simulink library "speedgoatlib_bce"  (R2024b)
settings: Solver=VariableStepAuto  StartTime=0.0  StopTime=10.0  RelTol=1e-3
undefined symbols (not defined in the file): BCE12, BCE_Set_init, Cell_1, Cell_10, Cell_11, Cell_12, Cell_2, Cell_3, Cell_4, Cell_5, Cell_6, Cell_7, Cell_8, Cell_9, Device_01, FIU12, sg_bce, TSE04
libraries: slrealtimeethercatlib x292, simulink x92, slrealtimeutilitieslib x24
(part 4 of 4)

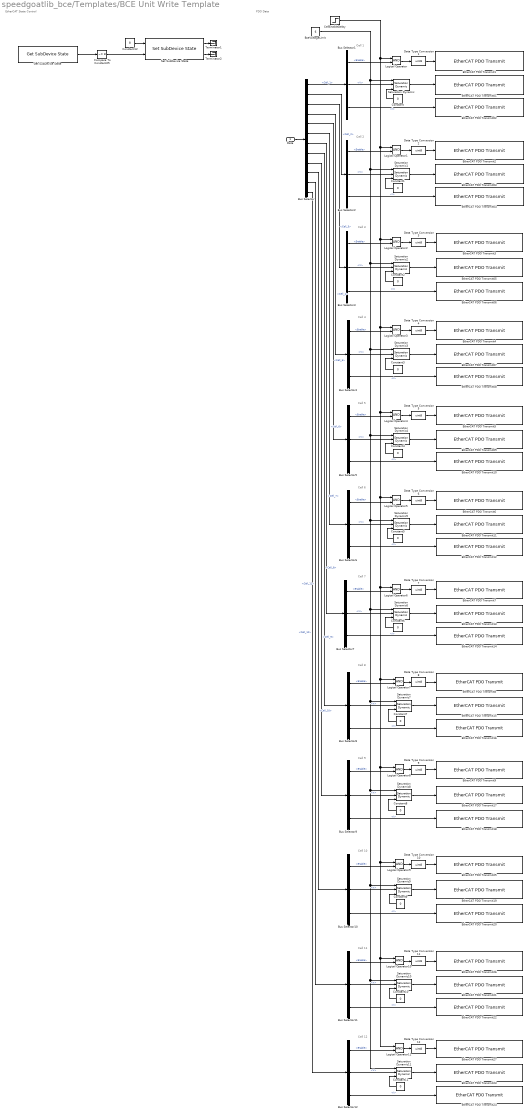
== system speedgoatlib_bce/Templates/BCE Unit Write Template  ==
  note: Cell 2
  note: Cell 12
  note: Cell 11
  note: Cell 6
  note: Cell 10
  note: Cell 3
  note: Cell 5
  note: PDO Data
  note: Cell 7
  note: Cell 1
  note: Cell 9
  note: Cell 8
  note: Cell 4
  note: EtherCAT State Control
  Data : Inport  OutDataTypeStr=Bus: BCE_Set
  BceVoltageLimit : Constant  Value=6
  Bus Selector : BusSelector  OutputSignals=Cell_1,Cell_2,Cell_3,Cell_4,Cell_5,Cell_6,Cell_7,Cell_8,Cell_9,Cell_10,Cell_11,Cell_12
  Bus Selector{1..12} (12 alike) : BusSelector  OutputSignals=Enable,V,I
  CellEnableDelay : Step  Time=2  SampleTime=0
  Compare To Constant25 : simulink/Logic and Bit Operations/Compare To Constant  relop=~=  const=8  OutDataTypeStr=boolean
  Constant{,1..11} (12 alike) : Constant  Value=0
  Constant12 : Constant  Value=8  OutDataTypeStr=int32
  Data Type Conversion{1..12} (12 alike) : DataTypeConversion  OutDataTypeStr=uint8  SaturateOnIntegerOverflow=off  RndMeth=Floor
  EtherCAT PDO Transmit01 : slrealtimeethercatlib/EtherCAT PDO Transmit  Priority=3  sig_name=Device_01 (BCE12-0605).Rx_Cell_01.setVoltage  sig_offset=8  sig_type=single  type_size=32  sig_dim=1  device_id=0  sample_time=0.001000
  EtherCAT PDO Transmit02 : slrealtimeethercatlib/EtherCAT PDO Transmit  Priority=3  sig_name=Device_01 (BCE12-0605).Rx_Cell_01.setCurrent  sig_offset=40  sig_type=single  type_size=32  sig_dim=1  device_id=0  sample_time=0.001000
  EtherCAT PDO Transmit03 : slrealtimeethercatlib/EtherCAT PDO Transmit  Priority=3  sig_name=Device_01 (BCE12-0605).Rx_Cell_02.setVoltage  sig_offset=80  sig_type=single  type_size=32  sig_dim=1  device_id=0  sample_time=0.001000
  EtherCAT PDO Transmit04 : slrealtimeethercatlib/EtherCAT PDO Transmit  Priority=3  sig_name=Device_01 (BCE12-0605).Rx_Cell_02.setCurrent  sig_offset=112  sig_type=single  type_size=32  sig_dim=1  device_id=0  sample_time=0.001000
  EtherCAT PDO Transmit05 : slrealtimeethercatlib/EtherCAT PDO Transmit  Priority=3  sig_name=Device_01 (BCE12-0605).Rx_Cell_03.setVoltage  sig_offset=152  sig_type=single  type_size=32  sig_dim=1  device_id=0  sample_time=0.001000
  EtherCAT PDO Transmit06 : slrealtimeethercatlib/EtherCAT PDO Transmit  Priority=3  sig_name=Device_01 (BCE12-0605).Rx_Cell_03.setCurrent  sig_offset=184  sig_type=single  type_size=32  sig_dim=1  device_id=0  sample_time=0.001000
  EtherCAT PDO Transmit07 : slrealtimeethercatlib/EtherCAT PDO Transmit  Priority=3  sig_name=Device_01 (BCE12-0605).Rx_Cell_04.setVoltage  sig_offset=224  sig_type=single  type_size=32  sig_dim=1  device_id=0  sample_time=0.001000
  EtherCAT PDO Transmit08 : slrealtimeethercatlib/EtherCAT PDO Transmit  Priority=3  sig_name=Device_01 (BCE12-0605).Rx_Cell_04.setCurrent  sig_offset=256  sig_type=single  type_size=32  sig_dim=1  device_id=0  sample_time=0.001000
  EtherCAT PDO Transmit09 : slrealtimeethercatlib/EtherCAT PDO Transmit  Priority=3  sig_name=Device_01 (BCE12-0605).Rx_Cell_05.setVoltage  sig_offset=296  sig_type=single  type_size=32  sig_dim=1  device_id=0  sample_time=0.001000
  EtherCAT PDO Transmit1 : slrealtimeethercatlib/EtherCAT PDO Transmit  Priority=3  sig_name=Device_01 (BCE12-0605).Rx_Cell_01.enableCell  sig_offset=0  sig_type=uint8  type_size=8  sig_dim=1  device_id=0  sample_time=0.001000
  EtherCAT PDO Transmit10 : slrealtimeethercatlib/EtherCAT PDO Transmit  Priority=3  sig_name=Device_01 (BCE12-0605).Rx_Cell_05.setCurrent  sig_offset=328  sig_type=single  type_size=32  sig_dim=1  device_id=0  sample_time=0.001000
  EtherCAT PDO Transmit11 : slrealtimeethercatlib/EtherCAT PDO Transmit  Priority=3  sig_name=Device_01 (BCE12-0605).Rx_Cell_06.setVoltage  sig_offset=368  sig_type=single  type_size=32  sig_dim=1  device_id=0  sample_time=0.001000
  EtherCAT PDO Transmit12 : slrealtimeethercatlib/EtherCAT PDO Transmit  Priority=3  sig_name=Device_01 (BCE12-0605).Rx_Cell_06.setCurrent  sig_offset=400  sig_type=single  type_size=32  sig_dim=1  device_id=0  sample_time=0.001000
  EtherCAT PDO Transmit13 : slrealtimeethercatlib/EtherCAT PDO Transmit  Priority=3  sig_name=Device_01 (BCE12-0605).Rx_Cell_07.setVoltage  sig_offset=440  sig_type=single  type_size=32  sig_dim=1  device_id=0  sample_time=0.001000
  EtherCAT PDO Transmit14 : slrealtimeethercatlib/EtherCAT PDO Transmit  Priority=3  sig_name=Device_01 (BCE12-0605).Rx_Cell_07.setCurrent  sig_offset=472  sig_type=single  type_size=32  sig_dim=1  device_id=0  sample_time=0.001000
  EtherCAT PDO Transmit15 : slrealtimeethercatlib/EtherCAT PDO Transmit  Priority=3  sig_name=Device_01 (BCE12-0605).Rx_Cell_08.setVoltage  sig_offset=512  sig_type=single  type_size=32  sig_dim=1  device_id=0  sample_time=0.001000
  EtherCAT PDO Transmit16 : slrealtimeethercatlib/EtherCAT PDO Transmit  Priority=3  sig_name=Device_01 (BCE12-0605).Rx_Cell_08.setCurrent  sig_offset=544  sig_type=single  type_size=32  sig_dim=1  device_id=0  sample_time=0.001000
  EtherCAT PDO Transmit17 : slrealtimeethercatlib/EtherCAT PDO Transmit  Priority=3  sig_name=Device_01 (BCE12-0605).Rx_Cell_09.setVoltage  sig_offset=584  sig_type=single  type_size=32  sig_dim=1  device_id=0  sample_time=0.001000
  EtherCAT PDO Transmit18 : slrealtimeethercatlib/EtherCAT PDO Transmit  Priority=3  sig_name=Device_01 (BCE12-0605).Rx_Cell_09.setCurrent  sig_offset=616  sig_type=single  type_size=32  sig_dim=1  device_id=0  sample_time=0.001000
  EtherCAT PDO Transmit19 : slrealtimeethercatlib/EtherCAT PDO Transmit  Priority=3  sig_name=Device_01 (BCE12-0605).Rx_Cell_10.setVoltage  sig_offset=656  sig_type=single  type_size=32  sig_dim=1  device_id=0  sample_time=0.001000
  EtherCAT PDO Transmit2 : slrealtimeethercatlib/EtherCAT PDO Transmit  Priority=3  sig_name=Device_01 (BCE12-0605).Rx_Cell_02.enableCell  sig_offset=72  sig_type=uint8  type_size=8  sig_dim=1  device_id=0  sample_time=0.001000
  EtherCAT PDO Transmit20 : slrealtimeethercatlib/EtherCAT PDO Transmit  Priority=3  sig_name=Device_01 (BCE12-0605).Rx_Cell_10.setCurrent  sig_offset=688  sig_type=single  type_size=32  sig_dim=1  device_id=0  sample_time=0.001000
  EtherCAT PDO Transmit21 : slrealtimeethercatlib/EtherCAT PDO Transmit  Priority=3  sig_name=Device_01 (BCE12-0605).Rx_Cell_11.setVoltage  sig_offset=728  sig_type=single  type_size=32  sig_dim=1  device_id=0  sample_time=0.001000
  EtherCAT PDO Transmit22 : slrealtimeethercatlib/EtherCAT PDO Transmit  Priority=3  sig_name=Device_01 (BCE12-0605).Rx_Cell_11.setCurrent  sig_offset=760  sig_type=single  type_size=32  sig_dim=1  device_id=0  sample_time=0.001000
  EtherCAT PDO Transmit23 : slrealtimeethercatlib/EtherCAT PDO Transmit  Priority=3  sig_name=Device_01 (BCE12-0605).Rx_Cell_12.setVoltage  sig_offset=800  sig_type=single  type_size=32  sig_dim=1  device_id=0  sample_time=0.001000
  EtherCAT PDO Transmit24 : slrealtimeethercatlib/EtherCAT PDO Transmit  Priority=3  sig_name=Device_01 (BCE12-0605).Rx_Cell_12.setCurrent  sig_offset=832  sig_type=single  type_size=32  sig_dim=1  device_id=0  sample_time=0.001000
  EtherCAT PDO Transmit25 : slrealtimeethercatlib/EtherCAT PDO Transmit  Priority=3  sig_name=Device_01 (BCE12-0605).Rx_Cell_10.enableCell  sig_offset=648  sig_type=uint8  type_size=8  sig_dim=1  device_id=0  sample_time=0.001000
  EtherCAT PDO Transmit26 : slrealtimeethercatlib/EtherCAT PDO Transmit  Priority=3  sig_name=Device_01 (BCE12-0605).Rx_Cell_11.enableCell  sig_offset=720  sig_type=uint8  type_size=8  sig_dim=1  device_id=0  sample_time=0.001000
  EtherCAT PDO Transmit27 : slrealtimeethercatlib/EtherCAT PDO Transmit  Priority=3  sig_name=Device_01 (BCE12-0605).Rx_Cell_12.enableCell  sig_offset=792  sig_type=uint8  type_size=8  sig_dim=1  device_id=0  sample_time=0.001000
  EtherCAT PDO Transmit3 : slrealtimeethercatlib/EtherCAT PDO Transmit  Priority=3  sig_name=Device_01 (BCE12-0605).Rx_Cell_03.enableCell  sig_offset=144  sig_type=uint8  type_size=8  sig_dim=1  device_id=0  sample_time=0.001000
  EtherCAT PDO Transmit4 : slrealtimeethercatlib/EtherCAT PDO Transmit  Priority=3  sig_name=Device_01 (BCE12-0605).Rx_Cell_04.enableCell  sig_offset=216  sig_type=uint8  type_size=8  sig_dim=1  device_id=0  sample_time=0.001000
  EtherCAT PDO Transmit5 : slrealtimeethercatlib/EtherCAT PDO Transmit  Priority=3  sig_name=Device_01 (BCE12-0605).Rx_Cell_05.enableCell  sig_offset=288  sig_type=uint8  type_size=8  sig_dim=1  device_id=0  sample_time=0.001000
  EtherCAT PDO Transmit6 : slrealtimeethercatlib/EtherCAT PDO Transmit  Priority=3  sig_name=Device_01 (BCE12-0605).Rx_Cell_06.enableCell  sig_offset=360  sig_type=uint8  type_size=8  sig_dim=1  device_id=0  sample_time=0.001000
  EtherCAT PDO Transmit7 : slrealtimeethercatlib/EtherCAT PDO Transmit  Priority=3  sig_name=Device_01 (BCE12-0605).Rx_Cell_07.enableCell  sig_offset=432  sig_type=uint8  type_size=8  sig_dim=1  device_id=0  sample_time=0.001000
  EtherCAT PDO Transmit8 : slrealtimeethercatlib/EtherCAT PDO Transmit  Priority=3  sig_name=Device_01 (BCE12-0605).Rx_Cell_08.enableCell  sig_offset=504  sig_type=uint8  type_size=8  sig_dim=1  device_id=0  sample_time=0.001000
  EtherCAT PDO Transmit9 : slrealtimeethercatlib/EtherCAT PDO Transmit  Priority=3  sig_name=Device_01 (BCE12-0605).Rx_Cell_09.enableCell  sig_offset=576  sig_type=uint8  type_size=8  sig_dim=1  device_id=0  sample_time=0.001000
  Get SubDevice State : slrealtimeethercatlib/Get SubDevice State  device_id=0  sample_time=1  subdevice_addr=0  selected_subdevice=Term 1 (EK1100)  timeout=500  subdevice_found=0
  Logical Operator{,1..11} (12 alike) : Logic  AllPortsSameDT=off  OutDataTypeStr=boolean
  Saturation Dynamic{,1..11} (12 alike) : simulink/Discontinuities/Saturation Dynamic  OutMin=[]  OutMax=[]  OutDataTypeStr=Inherit: Same as second input  OutDataType=fixdt(1, 16)  OutScaling=2^-10  DoSatur=off
  Set SubDevice State : slrealtimeethercatlib/Set SubDevice State  device_id=0  sample_time=1  subdevice_addr=0  selected_subdevice=Term 1 (EK1100)  subdevice_found=0
  Terminator1 : Terminator
  Terminator2 : Terminator
  wires:
  Data Type Conversion8/1 -> EtherCAT PDO Transmit8/1
  Bus Selector9/2 -> Saturation Dynamic8/2  "<V>"
  Bus Selector12/2 -> Saturation Dynamic11/2  "<V>"
  Bus Selector2/2 -> Saturation Dynamic1/2  "<V>"
  Bus Selector/7 -> Bus Selector7/1  "<Cell_7>"
  Bus Selector11/2 -> Saturation Dynamic10/2  "<V>"
  Bus Selector/1 -> Bus Selector1/1  "<Cell_1>"
  Bus Selector8/3 -> EtherCAT PDO Transmit16/1  "<I>"
  Bus Selector/3 -> Bus Selector3/1  "<Cell_3>"
  Bus Selector1/2 -> Saturation Dynamic/2  "<V>"
  Bus Selector/2 -> Bus Selector2/1  "<Cell_2>"
  Bus Selector/6 -> Bus Selector6/1  "<Cell_6>"
  Data Type Conversion2/1 -> EtherCAT PDO Transmit2/1
  Bus Selector7/2 -> Saturation Dynamic6/2  "<V>"
  Bus Selector7/3 -> EtherCAT PDO Transmit14/1  "<I>"
  Bus Selector/9 -> Bus Selector9/1  "<Cell_9>"
  Data Type Conversion4/1 -> EtherCAT PDO Transmit4/1
  Data Type Conversion6/1 -> EtherCAT PDO Transmit6/1
  Data Type Conversion9/1 -> EtherCAT PDO Transmit9/1
  Data Type Conversion5/1 -> EtherCAT PDO Transmit5/1
  Data Type Conversion12/1 -> EtherCAT PDO Transmit27/1
  Data Type Conversion10/1 -> EtherCAT PDO Transmit25/1
  Data Type Conversion1/1 -> EtherCAT PDO Transmit1/1
  Bus Selector4/3 -> EtherCAT PDO Transmit08/1  "<I>"
  Bus Selector/12 -> Bus Selector12/1  "<Cell_12>"
  Bus Selector3/3 -> EtherCAT PDO Transmit06/1  "<I>"
  Bus Selector6/2 -> Saturation Dynamic5/2  "<V>"
  Bus Selector4/2 -> Saturation Dynamic3/2  "<V>"
  Data Type Conversion3/1 -> EtherCAT PDO Transmit3/1
  Bus Selector1/3 -> EtherCAT PDO Transmit02/1  "<I>"
  Bus Selector/10 -> Bus Selector10/1  "<Cell_10>"
  Bus Selector/5 -> Bus Selector5/1  "<Cell_5>"
  Bus Selector12/3 -> EtherCAT PDO Transmit24/1  "<I>"
  Bus Selector10/2 -> Saturation Dynamic9/2  "<V>"
  Bus Selector2/3 -> EtherCAT PDO Transmit04/1  "<I>"
  Bus Selector3/2 -> Saturation Dynamic2/2  "<V>"
  Bus Selector/11 -> Bus Selector11/1  "<Cell_11>"
  Bus Selector10/3 -> EtherCAT PDO Transmit20/1  "<I>"
  Data/1 -> Bus Selector/1
  Bus Selector5/3 -> EtherCAT PDO Transmit10/1  "<I>"
  Data Type Conversion11/1 -> EtherCAT PDO Transmit26/1
  Bus Selector5/2 -> Saturation Dynamic4/2  "<V>"
  Bus Selector8/2 -> Saturation Dynamic7/2  "<V>"
  Bus Selector/8 -> Bus Selector8/1  "<Cell_8>"
  Bus Selector9/3 -> EtherCAT PDO Transmit18/1  "<I>"
  Bus Selector11/3 -> EtherCAT PDO Transmit22/1  "<I>"
  Data Type Conversion7/1 -> EtherCAT PDO Transmit7/1
  Bus Selector/4 -> Bus Selector4/1  "<Cell_4>"
  Bus Selector6/3 -> EtherCAT PDO Transmit12/1  "<I>"
  Saturation Dynamic/1 -> EtherCAT PDO Transmit01/1
  Constant/1 -> Saturation Dynamic/3
  BceVoltageLimit/1 -> Saturation Dynamic/1, Saturation Dynamic11/1, Saturation Dynamic10/1, Saturation Dynamic9/1, Saturation Dynamic8/1, Saturation Dynamic7/1, Saturation Dynamic6/1, Saturation Dynamic5/1, Saturation Dynamic4/1, Saturation Dynamic3/1, Saturation Dynamic2/1, Saturation Dynamic1/1
  Constant1/1 -> Saturation Dynamic1/3
  Saturation Dynamic1/1 -> EtherCAT PDO Transmit03/1
  Constant2/1 -> Saturation Dynamic2/3
  Saturation Dynamic2/1 -> EtherCAT PDO Transmit05/1
  Constant3/1 -> Saturation Dynamic3/3
  Saturation Dynamic3/1 -> EtherCAT PDO Transmit07/1
  Constant4/1 -> Saturation Dynamic4/3
  Saturation Dynamic4/1 -> EtherCAT PDO Transmit09/1
  Constant5/1 -> Saturation Dynamic5/3
  Saturation Dynamic5/1 -> EtherCAT PDO Transmit11/1
  Constant6/1 -> Saturation Dynamic6/3
  Saturation Dynamic6/1 -> EtherCAT PDO Transmit13/1
  Constant7/1 -> Saturation Dynamic7/3
  Saturation Dynamic7/1 -> EtherCAT PDO Transmit15/1
  Constant8/1 -> Saturation Dynamic8/3
  Saturation Dynamic8/1 -> EtherCAT PDO Transmit17/1
  Constant9/1 -> Saturation Dynamic9/3
  Saturation Dynamic9/1 -> EtherCAT PDO Transmit19/1
  Constant10/1 -> Saturation Dynamic10/3
  Saturation Dynamic10/1 -> EtherCAT PDO Transmit21/1
  Constant11/1 -> Saturation Dynamic11/3
  Saturation Dynamic11/1 -> EtherCAT PDO Transmit23/1
  Get SubDevice State/1 -> Compare To Constant25/1
  Set SubDevice State/2 -> Terminator2/1
  Set SubDevice State/1 -> Terminator1/1
  Compare To Constant25/1 -> Set SubDevice State/2
  Constant12/1 -> Set SubDevice State/1
  CellEnableDelay/1 -> Logical Operator11/1, Logical Operator10/1, Logical Operator9/1, Logical Operator8/1, Logical Operator7/1, Logical Operator6/1, Logical Operator5/1, Logical Operator4/1, Logical Operator3/1, Logical Operator2/1, Logical Operator1/1, Logical Operator/1
  Bus Selector1/1 -> Logical Operator/2  "<Enable>"
  Logical Operator/1 -> Data Type Conversion1/1
  Bus Selector2/1 -> Logical Operator1/2  "<Enable>"
  Logical Operator1/1 -> Data Type Conversion2/1
  Bus Selector3/1 -> Logical Operator2/2  "<Enable>"
  Logical Operator2/1 -> Data Type Conversion3/1
  Bus Selector4/1 -> Logical Operator3/2  "<Enable>"
  Logical Operator3/1 -> Data Type Conversion4/1
  Bus Selector5/1 -> Logical Operator4/2  "<Enable>"
  Logical Operator4/1 -> Data Type Conversion5/1
  Bus Selector6/1 -> Logical Operator5/2  "<Enable>"
  Logical Operator5/1 -> Data Type Conversion6/1
  Bus Selector7/1 -> Logical Operator6/2  "<Enable>"
  Logical Operator6/1 -> Data Type Conversion7/1
  Bus Selector8/1 -> Logical Operator7/2  "<Enable>"
  Logical Operator7/1 -> Data Type Conversion8/1
  Bus Selector9/1 -> Logical Operator8/2  "<Enable>"
  Logical Operator8/1 -> Data Type Conversion9/1
  Bus Selector10/1 -> Logical Operator9/2  "<Enable>"
  Logical Operator9/1 -> Data Type Conversion10/1
  Bus Selector11/1 -> Logical Operator10/2  "<Enable>"
  Logical Operator10/1 -> Data Type Conversion11/1
  Bus Selector12/1 -> Logical Operator11/2  "<Enable>"
  Logical Operator11/1 -> Data Type Conversion12/1

== system speedgoatlib_bce/Templates/FIU Channel Read Template  ==
  note: Channel X
  Bus Creator : BusCreator  Inputs=1  OutDataTypeStr=Bus: FIU_Get
      settings: InheritFromInputs=off
  EtherCAT PDO Receive01 : slrealtimeethercatlib/EtherCAT PDO Receive  Priority=2  sig_name=Device_01 (FIU12-1).Tx_Channel_01.status  sig_offset=0  sig_type=uint8  type_size=8  sig_dim=1  device_id=0  sample_time=0.001000
  Data : Outport  OutDataTypeStr=Bus: FIU_Get
  wires:
  EtherCAT PDO Receive01/1 -> Bus Creator/1  "ChX_Status"
  Bus Creator/1 -> Data/1

== system speedgoatlib_bce/Templates/FIU Channel Write Template  ==
  note: Update
  Data : Inport  OutDataTypeStr=Bus: FIU_Set
  Add : Sum  Inputs=+++
  Bus Selector : BusSelector  OutputSignals=FaultState,SensePlusBroken,SenseMinusBroken
  Constant3 : Constant  Value=8  OutDataTypeStr=uint8
  Constant4 : Constant  Value=0  OutDataTypeStr=uint8
  Constant6 : Constant  Value=16  OutDataTypeStr=uint8
  Constant7 : Constant  Value=0  OutDataTypeStr=uint8
  EtherCAT PDO Transmit02 : slrealtimeethercatlib/EtherCAT PDO Transmit  Priority=3  sig_name=Device_01 (FIU12-1).Rx_Channel_01.faultState  sig_offset=8  sig_type=uint8  type_size=8  sig_dim=1  device_id=0  sample_time=0.001000
  EtherCAT State Control : Subsystem
  Range Assert : MATLAB Function  TreatAsAtomicUnit=on
  Switch : Switch  Criteria=u2 > Threshold  SaturateOnIntegerOverflow=off  InputSameDT=off
  Switch1 : Switch  Criteria=u2 > Threshold  SaturateOnIntegerOverflow=off  InputSameDT=off
  wires:
  Bus Selector/1 -> Range Assert/1(u)  "<FaultState>"
  Switch1/1 -> Add/3
  Bus Selector/3 -> Switch1/2  "<SenseMinusBroken>"
  Add/1 -> EtherCAT PDO Transmit02/1
  Constant7/1 -> Switch1/3
  Constant4/1 -> Switch/3
  Switch/1 -> Add/2
  Constant3/1 -> Switch/1
  Constant6/1 -> Switch1/1
  Bus Selector/2 -> Switch/2  "<SensePlusBroken>"
  Data/1 -> Bus Selector/1
  Range Assert/1(y) -> Add/1

== system speedgoatlib_bce/Templates/TSE Channel Read Template  ==
  note: Channel X
  Bus Creator : BusCreator  Inputs=1  OutDataTypeStr=Bus: TSE_Get
      settings: InheritFromInputs=off
  EtherCAT PDO Receive01 : slrealtimeethercatlib/EtherCAT PDO Receive  Priority=2  sig_name=Device_01 (TSE04-1000-1).Tx_Channel_01.status  sig_offset=0  sig_type=single  type_size=32  sig_dim=1  device_id=0  sample_time=0.001000
  Data : Outport  OutDataTypeStr=Bus: TSE_Get
  wires:
  EtherCAT PDO Receive01/1 -> Bus Creator/1  "ChX_Status"
  Bus Creator/1 -> Data/1

== system speedgoatlib_bce/Templates/TSE Channel Write Template  ==
  note: Update
  Data : Inport  OutDataTypeStr=Bus: TSE_Set
  Bus Selector : BusSelector  OutputSignals=Resistance
  EtherCAT PDO Transmit02 : slrealtimeethercatlib/EtherCAT PDO Transmit  Priority=3  sig_name=Device_01 (TSE04-1000-1).Rx_Channel_01.resistance  sig_offset=8  sig_type=double  type_size=64  sig_dim=1  device_id=0  sample_time=0.001000
  EtherCAT State Control : Subsystem
  wires:
  Data/1 -> Bus Selector/1
  Bus Selector/1 -> EtherCAT PDO Transmit02/1  "<Resistance>"

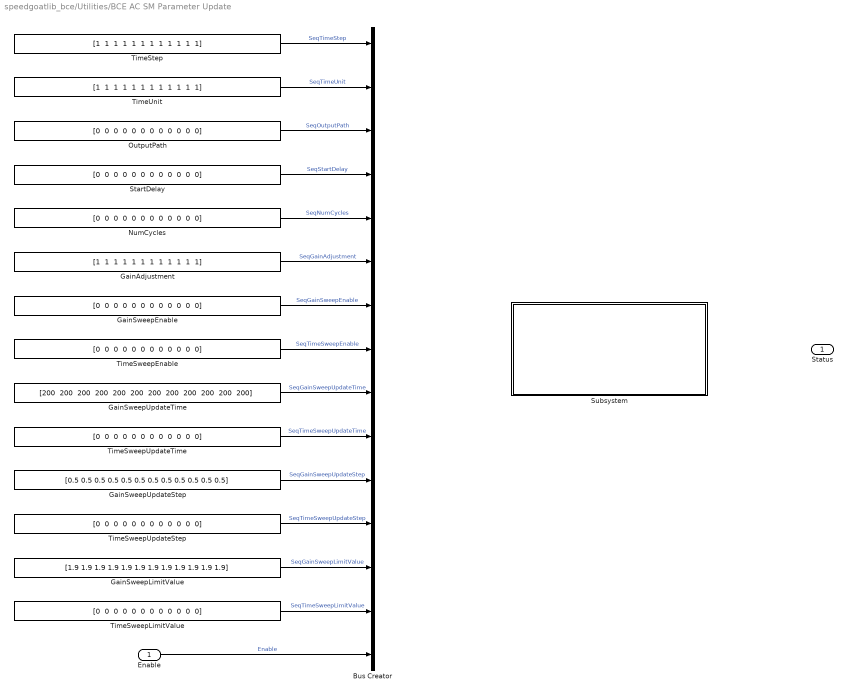
== system speedgoatlib_bce/Utilities/BCE AC SM Parameter Update  ==
  Enable : Inport  OutDataTypeStr=boolean
  Bus Creator : BusCreator  Inputs=15
  GainAdjustment : Constant  Value="[1  1  1  1  1  1  1  1  1  1  1  1]"  OutDataTypeStr=double
  GainSweepEnable : Constant  Value="[0  0  0  0  0  0  0  0  0  0  0  0]"  OutDataTypeStr=boolean
  GainSweepLimitValue : Constant  Value="[1.9         1.9         1.9         1.9         1.9         1.9         1.9         1.9         1.9         1.9         1.9         1.9]"  OutDataTypeStr=double
  GainSweepUpdateStep : Constant  Value="[0.5         0.5         0.5         0.5         0.5         0.5         0.5         0.5         0.5         0.5         0.5         0.5]"  OutDataTypeStr=double
  GainSweepUpdateTime : Constant  Value="[200  200  200  200  200  200  200  200  200  200  200  200]"  OutDataTypeStr=uint16
  NumCycles : Constant  Value="[0  0  0  0  0  0  0  0  0  0  0  0]"  OutDataTypeStr=uint16
  OutputPath : Constant  Value="[0  0  0  0  0  0  0  0  0  0  0  0]"  OutDataTypeStr=boolean
  StartDelay : Constant  Value="[0  0  0  0  0  0  0  0  0  0  0  0]"  OutDataTypeStr=uint16
  Subsystem : Subsystem
  TimeStep : Constant  Value="[1  1  1  1  1  1  1  1  1  1  1  1]"  OutDataTypeStr=uint16
  TimeSweepEnable : Constant  Value="[0  0  0  0  0  0  0  0  0  0  0  0]"  OutDataTypeStr=boolean
  TimeSweepLimitValue : Constant  Value="[0  0  0  0  0  0  0  0  0  0  0  0]"  OutDataTypeStr=uint16
  TimeSweepUpdateStep : Constant  Value="[0  0  0  0  0  0  0  0  0  0  0  0]"  OutDataTypeStr=uint16
  TimeSweepUpdateTime : Constant  Value="[0  0  0  0  0  0  0  0  0  0  0  0]"  OutDataTypeStr=uint16
  TimeUnit : Constant  Value="[1  1  1  1  1  1  1  1  1  1  1  1]"  OutDataTypeStr=boolean
  Status : Outport
  wires:
  GainSweepLimitValue/1 -> Bus Creator/13  "SeqGainSweepLimitValue"
  TimeSweepUpdateStep/1 -> Bus Creator/12  "SeqTimeSweepUpdateStep"
  GainSweepUpdateStep/1 -> Bus Creator/11  "SeqGainSweepUpdateStep"
  TimeSweepLimitValue/1 -> Bus Creator/14  "SeqTimeSweepLimitValue"
  TimeSweepUpdateTime/1 -> Bus Creator/10  "SeqTimeSweepUpdateTime"
  GainSweepUpdateTime/1 -> Bus Creator/9  "SeqGainSweepUpdateTime"
  TimeStep/1 -> Bus Creator/1  "SeqTimeStep"
  OutputPath/1 -> Bus Creator/3  "SeqOutputPath"
  TimeSweepEnable/1 -> Bus Creator/8  "SeqTimeSweepEnable"
  StartDelay/1 -> Bus Creator/4  "SeqStartDelay"
  GainSweepEnable/1 -> Bus Creator/7  "SeqGainSweepEnable"
  TimeUnit/1 -> Bus Creator/2  "SeqTimeUnit"
  NumCycles/1 -> Bus Creator/5  "SeqNumCycles"
  GainAdjustment/1 -> Bus Creator/6  "SeqGainAdjustment"
  Enable/1 -> Bus Creator/15  "Enable"

== system speedgoatlib_bce/Utilities/BMTS Bus Pack  ==
  Cell_1.Enable : Inport
  Cell_2.Enable : Inport  Port=2
  Cell_1.V : Inport  Port=3
  Cell_2.V : Inport  Port=4
  Cell_1.I : Inport  Port=5
  Cell_2.I : Inport  Port=6
  Bus Assignment : BusAssignment  AssignedSignals=Cell_1.Enable,Cell_2.Enable,Cell_1.V,Cell_2.V,Cell_1.I,Cell_2.I
  Bus Structure : Constant  Value=BCE_Set_init  OutDataTypeStr=Bus: BCE_Set
  Bus : Outport
  wires:
  Bus Structure/1 -> Bus Assignment/1
  Cell_1.I/1 -> Bus Assignment/6
  Cell_1.V/1 -> Bus Assignment/4
  Cell_1.Enable/1 -> Bus Assignment/2
  Bus Assignment/1 -> Bus/1
  Cell_2.I/1 -> Bus Assignment/7
  Cell_2.V/1 -> Bus Assignment/5
  Cell_2.Enable/1 -> Bus Assignment/3

== system speedgoatlib_bce/Templates/BCE AC SM Parameter Update Template /Enabled Subsystem ==
  Enable : EnablePort  StatesWhenEnabling=reset
  Add : Sum
  Compare To Constant : simulink/Logic and Bit Operations/Compare To Constant  relop=>=  const=2  OutDataTypeStr=boolean
  Constant : Constant
  Unit Delay : UnitDelay  SampleTime=-1
  Out1 : Outport  OutputWhenDisabled=reset  InitialOutput=0
  wires:
  Compare To Constant/1 -> Out1/1
  Add/1 -> Unit Delay/1, Compare To Constant/1
  Constant/1 -> Add/1
  Unit Delay/1 -> Add/2

== system speedgoatlib_bce/Templates/BCE AC SM Parameter Update Template /Enabled Subsystem1 ==
  Enable : EnablePort  StatesWhenEnabling=reset
  Add : Sum
  Compare To Constant : simulink/Logic and Bit Operations/Compare To Constant  relop=>=  const=2  OutDataTypeStr=boolean
  Constant : Constant
  Unit Delay : UnitDelay  SampleTime=-1
  Out1 : Outport  OutputWhenDisabled=reset  InitialOutput=0
  wires:
  Add/1 -> Unit Delay/1, Compare To Constant/1
  Constant/1 -> Add/1
  Compare To Constant/1 -> Out1/1
  Unit Delay/1 -> Add/2

== system speedgoatlib_bce/Templates/BCE AC SM Parameter Update Template /Enabled Subsystem10 ==
  Enable : EnablePort  StatesWhenEnabling=reset
  Add : Sum
  Compare To Constant : simulink/Logic and Bit Operations/Compare To Constant  relop=>=  const=2  OutDataTypeStr=boolean
  Constant : Constant
  Unit Delay : UnitDelay  SampleTime=-1
  Out1 : Outport  OutputWhenDisabled=reset  InitialOutput=0
  wires:
  Unit Delay/1 -> Add/2
  Compare To Constant/1 -> Out1/1
  Constant/1 -> Add/1
  Add/1 -> Compare To Constant/1, Unit Delay/1

== system speedgoatlib_bce/Templates/BCE AC SM Parameter Update Template /Enabled Subsystem11 ==
  Enable : EnablePort  StatesWhenEnabling=reset
  Add : Sum
  Compare To Constant : simulink/Logic and Bit Operations/Compare To Constant  relop=>=  const=2  OutDataTypeStr=boolean
  Constant : Constant
  Display : Display
  Unit Delay : UnitDelay  SampleTime=-1
  Out1 : Outport  OutputWhenDisabled=reset  InitialOutput=0
  wires:
  Add/1 -> Unit Delay/1, Display/1, Compare To Constant/1
  Constant/1 -> Add/1
  Compare To Constant/1 -> Out1/1
  Unit Delay/1 -> Add/2

== system speedgoatlib_bce/Templates/BCE AC SM Parameter Update Template /Enabled Subsystem2 ==
  Enable : EnablePort  StatesWhenEnabling=reset
  Add : Sum
  Compare To Constant : simulink/Logic and Bit Operations/Compare To Constant  relop=>=  const=2  OutDataTypeStr=boolean
  Constant : Constant
  Unit Delay : UnitDelay  SampleTime=-1
  Out1 : Outport  OutputWhenDisabled=reset  InitialOutput=0
  wires:
  Unit Delay/1 -> Add/2
  Compare To Constant/1 -> Out1/1
  Constant/1 -> Add/1
  Add/1 -> Compare To Constant/1, Unit Delay/1

== system speedgoatlib_bce/Templates/BCE AC SM Parameter Update Template /Enabled Subsystem3 ==
  Enable : EnablePort  StatesWhenEnabling=reset
  Add : Sum
  Compare To Constant : simulink/Logic and Bit Operations/Compare To Constant  relop=>=  const=2  OutDataTypeStr=boolean
  Constant : Constant
  Unit Delay : UnitDelay  SampleTime=-1
  Out1 : Outport  OutputWhenDisabled=reset  InitialOutput=0
  wires:
  Add/1 -> Unit Delay/1, Compare To Constant/1
  Constant/1 -> Add/1
  Compare To Constant/1 -> Out1/1
  Unit Delay/1 -> Add/2

== system speedgoatlib_bce/Templates/BCE AC SM Parameter Update Template /Enabled Subsystem4 ==
  Enable : EnablePort  StatesWhenEnabling=reset
  Add : Sum
  Compare To Constant : simulink/Logic and Bit Operations/Compare To Constant  relop=>=  const=2  OutDataTypeStr=boolean
  Constant : Constant
  Unit Delay : UnitDelay  SampleTime=-1
  Out1 : Outport  OutputWhenDisabled=reset  InitialOutput=0
  wires:
  Unit Delay/1 -> Add/2
  Compare To Constant/1 -> Out1/1
  Constant/1 -> Add/1
  Add/1 -> Compare To Constant/1, Unit Delay/1

== system speedgoatlib_bce/Templates/BCE AC SM Parameter Update Template /Enabled Subsystem5 ==
  Enable : EnablePort  StatesWhenEnabling=reset
  Add : Sum
  Compare To Constant : simulink/Logic and Bit Operations/Compare To Constant  relop=>=  const=2  OutDataTypeStr=boolean
  Constant : Constant
  Unit Delay : UnitDelay  SampleTime=-1
  Out1 : Outport  OutputWhenDisabled=reset  InitialOutput=0
  wires:
  Add/1 -> Unit Delay/1, Compare To Constant/1
  Constant/1 -> Add/1
  Compare To Constant/1 -> Out1/1
  Unit Delay/1 -> Add/2

== system speedgoatlib_bce/Templates/BCE AC SM Parameter Update Template /Enabled Subsystem6 ==
  Enable : EnablePort  StatesWhenEnabling=reset
  Add : Sum
  Compare To Constant : simulink/Logic and Bit Operations/Compare To Constant  relop=>=  const=2  OutDataTypeStr=boolean
  Constant : Constant
  Unit Delay : UnitDelay  SampleTime=-1
  Out1 : Outport  OutputWhenDisabled=reset  InitialOutput=0
  wires:
  Unit Delay/1 -> Add/2
  Compare To Constant/1 -> Out1/1
  Constant/1 -> Add/1
  Add/1 -> Compare To Constant/1, Unit Delay/1

== system speedgoatlib_bce/Templates/BCE AC SM Parameter Update Template /Enabled Subsystem7 ==
  Enable : EnablePort  StatesWhenEnabling=reset
  Add : Sum
  Compare To Constant : simulink/Logic and Bit Operations/Compare To Constant  relop=>=  const=2  OutDataTypeStr=boolean
  Constant : Constant
  Unit Delay : UnitDelay  SampleTime=-1
  Out1 : Outport  OutputWhenDisabled=reset  InitialOutput=0
  wires:
  Add/1 -> Unit Delay/1, Compare To Constant/1
  Constant/1 -> Add/1
  Compare To Constant/1 -> Out1/1
  Unit Delay/1 -> Add/2

== system speedgoatlib_bce/Templates/BCE AC SM Parameter Update Template /Enabled Subsystem8 ==
  Enable : EnablePort  StatesWhenEnabling=reset
  Add : Sum
  Compare To Constant : simulink/Logic and Bit Operations/Compare To Constant  relop=>=  const=2  OutDataTypeStr=boolean
  Constant : Constant
  Unit Delay : UnitDelay  SampleTime=-1
  Out1 : Outport  OutputWhenDisabled=reset  InitialOutput=0
  wires:
  Unit Delay/1 -> Add/2
  Compare To Constant/1 -> Out1/1
  Constant/1 -> Add/1
  Add/1 -> Compare To Constant/1, Unit Delay/1

== system speedgoatlib_bce/Templates/BCE AC SM Parameter Update Template /Enabled Subsystem9 ==
  Enable : EnablePort  StatesWhenEnabling=reset
  Add : Sum
  Compare To Constant : simulink/Logic and Bit Operations/Compare To Constant  relop=>=  const=2  OutDataTypeStr=boolean
  Constant : Constant
  Unit Delay : UnitDelay  SampleTime=-1
  Out1 : Outport  OutputWhenDisabled=reset  InitialOutput=0
  wires:
  Add/1 -> Unit Delay/1, Compare To Constant/1
  Constant/1 -> Add/1
  Compare To Constant/1 -> Out1/1
  Unit Delay/1 -> Add/2

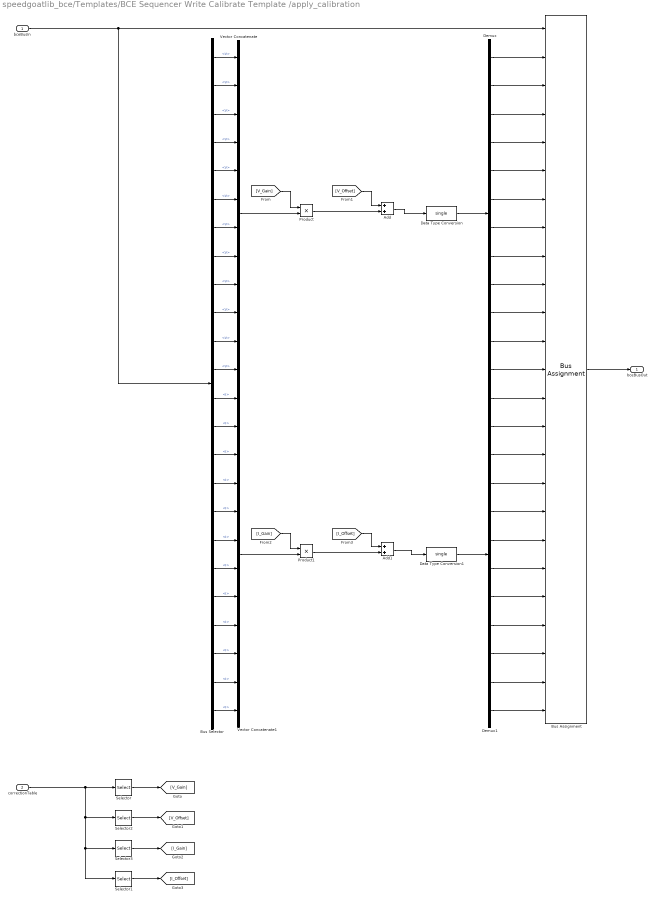
== system speedgoatlib_bce/Templates/BCE Sequencer Write Calibrate Template /apply_calibration ==
  bceBusIn : Inport  OutDataTypeStr=Bus: BCE_Set
  correctionTable : Inport  Port=2  PortDimensions=[12, 4]
  Add : Sum
  Add1 : Sum
  Bus Assignment : BusAssignment  AssignedSignals=Cell_1.V,Cell_2.V,Cell_3.V,Cell_4.V,Cell_5.V,Cell_6.V,Cell_7.V,Cell_8.V,Cell_9.V,Cell_10.V,Cell_11.V,Cell_12.V,Cell_1.I,Cell_2.I,Cell_3.I,Cell_4.I,Cell_5.I,Cell_6.I,Cell_7.I,Cell_8.I,Cell_9.I,Cell_10.I,Cell_11.I,Cell_12.I
  Bus Selector : BusSelector  OutputSignals=Cell_1.V,Cell_2.V,Cell_3.V,Cell_4.V,Cell_5.V,Cell_6.V,Cell_7.V,Cell_8.V,Cell_9.V,Cell_10.V,Cell_11.V,Cell_12.V,Cell_1.I,Cell_2.I,Cell_3.I,Cell_4.I,Cell_5.I,Cell_6.I,Cell_7.I,Cell_8.I,Cell_9.I,Cell_10.I,Cell_11.I,Cell_12.I
  Data Type Conversion : DataTypeConversion  OutDataTypeStr=single  SaturateOnIntegerOverflow=off  RndMeth=Floor
  Data Type Conversion1 : DataTypeConversion  OutDataTypeStr=single  SaturateOnIntegerOverflow=off  RndMeth=Floor
  Demux : Demux  Outputs=12
  Demux1 : Demux  Outputs=12
  Product : Product
  Product1 : Product
  Selector : Selector  NumberOfDimensions=2  InputPortWidth=3  IndexOptions=Select all,Index vector (dialog)  Indices=1,1  OutputSizes=1,1
  Selector1 : Selector  NumberOfDimensions=2  InputPortWidth=3  IndexOptions=Select all,Index vector (dialog)  Indices=4,4  OutputSizes=1,1
  Selector2 : Selector  NumberOfDimensions=2  InputPortWidth=3  IndexOptions=Select all,Index vector (dialog)  Indices=2,2  OutputSizes=1,1
  Selector3 : Selector  NumberOfDimensions=2  InputPortWidth=3  IndexOptions=Select all,Index vector (dialog)  Indices=3,3  OutputSizes=1,1
  Vector Concatenate : Concatenate  NumInputs=12
  Vector Concatenate1 : Concatenate  NumInputs=12
  bceBusOut : Outport  OutDataTypeStr=Bus: BCE_Set
  wires:
  bceBusIn/1 -> Bus Selector/1, Bus Assignment/1
  correctionTable/1 -> Selector3/1, Selector1/1, Selector2/1, Selector/1
  Bus Assignment/1 -> bceBusOut/1
  Bus Selector/1 -> Vector Concatenate/1  "<V>"
  Bus Selector/2 -> Vector Concatenate/2  "<V>"
  Bus Selector/3 -> Vector Concatenate/3  "<V>"
  Bus Selector/4 -> Vector Concatenate/4  "<V>"
  Bus Selector/5 -> Vector Concatenate/5  "<V>"
  Bus Selector/6 -> Vector Concatenate/6  "<V>"
  Bus Selector/7 -> Vector Concatenate/7  "<V>"
  Bus Selector/8 -> Vector Concatenate/8  "<V>"
  Bus Selector/9 -> Vector Concatenate/9  "<V>"
  Bus Selector/10 -> Vector Concatenate/10  "<V>"
  Bus Selector/11 -> Vector Concatenate/11  "<V>"
  Bus Selector/12 -> Vector Concatenate/12  "<V>"
  Vector Concatenate/1 -> Product/2
  Product/1 -> Add/2
  Demux/7 -> Bus Assignment/8
  Demux/6 -> Bus Assignment/7
  Demux/8 -> Bus Assignment/9
  Demux/5 -> Bus Assignment/6
  Demux/9 -> Bus Assignment/10
  Demux/4 -> Bus Assignment/5
  Demux/10 -> Bus Assignment/11
  Demux/3 -> Bus Assignment/4
  Demux/11 -> Bus Assignment/12
  Demux/2 -> Bus Assignment/3
  Demux/12 -> Bus Assignment/13
  Demux/1 -> Bus Assignment/2
  Add/1 -> Data Type Conversion/1
  Add1/1 -> Data Type Conversion1/1
  Demux1/1 -> Bus Assignment/14
  Demux1/12 -> Bus Assignment/25
  Demux1/2 -> Bus Assignment/15
  Demux1/11 -> Bus Assignment/24
  Demux1/3 -> Bus Assignment/16
  Demux1/10 -> Bus Assignment/23
  Demux1/4 -> Bus Assignment/17
  Demux1/9 -> Bus Assignment/22
  Demux1/5 -> Bus Assignment/18
  Demux1/8 -> Bus Assignment/21
  Demux1/6 -> Bus Assignment/19
  Demux1/7 -> Bus Assignment/20
  Product1/1 -> Add1/2
  Vector Concatenate1/1 -> Product1/2
  Bus Selector/24 -> Vector Concatenate1/12  "<I>"
  Bus Selector/23 -> Vector Concatenate1/11  "<I>"
  Bus Selector/22 -> Vector Concatenate1/10  "<I>"
  Bus Selector/21 -> Vector Concatenate1/9  "<I>"
  Bus Selector/20 -> Vector Concatenate1/8  "<I>"
  Bus Selector/19 -> Vector Concatenate1/7  "<I>"
  Bus Selector/18 -> Vector Concatenate1/6  "<I>"
  Bus Selector/17 -> Vector Concatenate1/5  "<I>"
  Bus Selector/16 -> Vector Concatenate1/4  "<I>"
  Bus Selector/15 -> Vector Concatenate1/3  "<I>"
  Bus Selector/14 -> Vector Concatenate1/2  "<I>"
  Bus Selector/13 -> Vector Concatenate1/1  "<I>"
  Selector/1 -> [V_Gain]
  Selector2/1 -> [V_Offset]
  Selector3/1 -> [I_Gain]
  Selector1/1 -> [I_Offset]
  [V_Gain] -> Product/1
  [V_Offset] -> Add/1
  [I_Gain] -> Product1/1
  [I_Offset] -> Add1/1
  Data Type Conversion/1 -> Demux/1
  Data Type Conversion1/1 -> Demux1/1

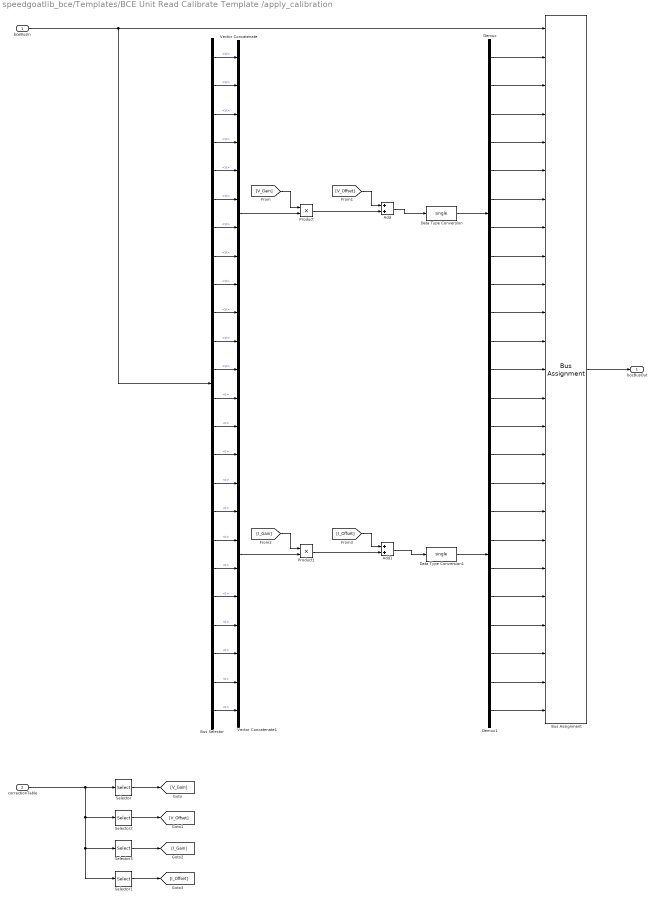
== system speedgoatlib_bce/Templates/BCE Unit Read Calibrate Template /apply_calibration ==
  bceBusIn : Inport  OutDataTypeStr=Bus: BCE_Get
  correctionTable : Inport  Port=2  PortDimensions=[12, 4]
  Add : Sum
  Add1 : Sum
  Bus Assignment : BusAssignment  AssignedSignals=Cell_1.V,Cell_2.V,Cell_3.V,Cell_4.V,Cell_5.V,Cell_6.V,Cell_7.V,Cell_8.V,Cell_9.V,Cell_10.V,Cell_11.V,Cell_12.V,Cell_1.I,Cell_2.I,Cell_3.I,Cell_4.I,Cell_5.I,Cell_6.I,Cell_7.I,Cell_8.I,Cell_9.I,Cell_10.I,Cell_11.I,Cell_12.I
  Bus Selector : BusSelector  OutputSignals=Cell_1.V,Cell_2.V,Cell_3.V,Cell_4.V,Cell_5.V,Cell_6.V,Cell_7.V,Cell_8.V,Cell_9.V,Cell_10.V,Cell_11.V,Cell_12.V,Cell_1.I,Cell_2.I,Cell_3.I,Cell_4.I,Cell_5.I,Cell_6.I,Cell_7.I,Cell_8.I,Cell_9.I,Cell_10.I,Cell_11.I,Cell_12.I
  Data Type Conversion : DataTypeConversion  OutDataTypeStr=single  SaturateOnIntegerOverflow=off  RndMeth=Floor
  Data Type Conversion1 : DataTypeConversion  OutDataTypeStr=single  SaturateOnIntegerOverflow=off  RndMeth=Floor
  Demux : Demux  Outputs=12
  Demux1 : Demux  Outputs=12
  Product : Product
  Product1 : Product
  Selector : Selector  NumberOfDimensions=2  InputPortWidth=3  IndexOptions=Select all,Index vector (dialog)  Indices=1,1  OutputSizes=1,1
  Selector1 : Selector  NumberOfDimensions=2  InputPortWidth=3  IndexOptions=Select all,Index vector (dialog)  Indices=4,4  OutputSizes=1,1
  Selector2 : Selector  NumberOfDimensions=2  InputPortWidth=3  IndexOptions=Select all,Index vector (dialog)  Indices=2,2  OutputSizes=1,1
  Selector3 : Selector  NumberOfDimensions=2  InputPortWidth=3  IndexOptions=Select all,Index vector (dialog)  Indices=3,3  OutputSizes=1,1
  Vector Concatenate : Concatenate  NumInputs=12
  Vector Concatenate1 : Concatenate  NumInputs=12
  bceBusOut : Outport  OutDataTypeStr=Bus: BCE_Get
  wires:
  bceBusIn/1 -> Bus Selector/1, Bus Assignment/1
  correctionTable/1 -> Selector3/1, Selector1/1, Selector2/1, Selector/1
  Bus Assignment/1 -> bceBusOut/1
  Bus Selector/1 -> Vector Concatenate/1  "<V>"
  Bus Selector/2 -> Vector Concatenate/2  "<V>"
  Bus Selector/3 -> Vector Concatenate/3  "<V>"
  Bus Selector/4 -> Vector Concatenate/4  "<V>"
  Bus Selector/5 -> Vector Concatenate/5  "<V>"
  Bus Selector/6 -> Vector Concatenate/6  "<V>"
  Bus Selector/7 -> Vector Concatenate/7  "<V>"
  Bus Selector/8 -> Vector Concatenate/8  "<V>"
  Bus Selector/9 -> Vector Concatenate/9  "<V>"
  Bus Selector/10 -> Vector Concatenate/10  "<V>"
  Bus Selector/11 -> Vector Concatenate/11  "<V>"
  Bus Selector/12 -> Vector Concatenate/12  "<V>"
  Vector Concatenate/1 -> Product/2
  Product/1 -> Add/2
  Demux/7 -> Bus Assignment/8
  Demux/6 -> Bus Assignment/7
  Demux/8 -> Bus Assignment/9
  Demux/5 -> Bus Assignment/6
  Demux/9 -> Bus Assignment/10
  Demux/4 -> Bus Assignment/5
  Demux/10 -> Bus Assignment/11
  Demux/3 -> Bus Assignment/4
  Demux/11 -> Bus Assignment/12
  Demux/2 -> Bus Assignment/3
  Demux/12 -> Bus Assignment/13
  Demux/1 -> Bus Assignment/2
  Add/1 -> Data Type Conversion/1
  Add1/1 -> Data Type Conversion1/1
  Demux1/1 -> Bus Assignment/14
  Demux1/12 -> Bus Assignment/25
  Demux1/2 -> Bus Assignment/15
  Demux1/11 -> Bus Assignment/24
  Demux1/3 -> Bus Assignment/16
  Demux1/10 -> Bus Assignment/23
  Demux1/4 -> Bus Assignment/17
  Demux1/9 -> Bus Assignment/22
  Demux1/5 -> Bus Assignment/18
  Demux1/8 -> Bus Assignment/21
  Demux1/6 -> Bus Assignment/19
  Demux1/7 -> Bus Assignment/20
  Product1/1 -> Add1/2
  Vector Concatenate1/1 -> Product1/2
  Bus Selector/24 -> Vector Concatenate1/12  "<I>"
  Bus Selector/23 -> Vector Concatenate1/11  "<I>"
  Bus Selector/22 -> Vector Concatenate1/10  "<I>"
  Bus Selector/21 -> Vector Concatenate1/9  "<I>"
  Bus Selector/20 -> Vector Concatenate1/8  "<I>"
  Bus Selector/19 -> Vector Concatenate1/7  "<I>"
  Bus Selector/18 -> Vector Concatenate1/6  "<I>"
  Bus Selector/17 -> Vector Concatenate1/5  "<I>"
  Bus Selector/16 -> Vector Concatenate1/4  "<I>"
  Bus Selector/15 -> Vector Concatenate1/3  "<I>"
  Bus Selector/14 -> Vector Concatenate1/2  "<I>"
  Bus Selector/13 -> Vector Concatenate1/1  "<I>"
  Selector/1 -> [V_Gain]
  Selector2/1 -> [V_Offset]
  Selector3/1 -> [I_Gain]
  Selector1/1 -> [I_Offset]
  [V_Gain] -> Product/1
  [V_Offset] -> Add/1
  [I_Gain] -> Product1/1
  [I_Offset] -> Add1/1
  Data Type Conversion/1 -> Demux/1
  Data Type Conversion1/1 -> Demux1/1

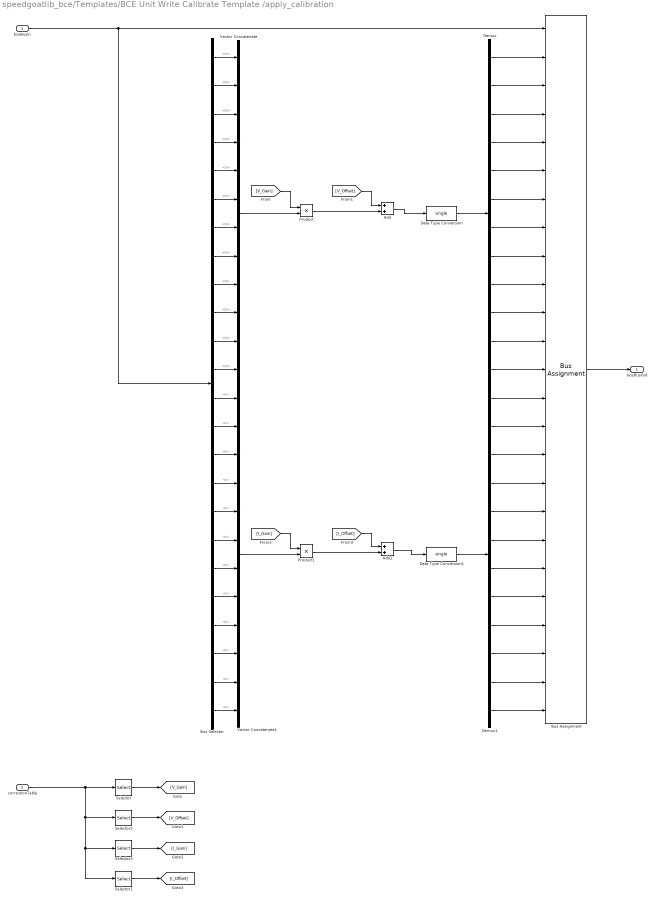
== system speedgoatlib_bce/Templates/BCE Unit Write Calibrate Template /apply_calibration ==
  bceBusIn : Inport  OutDataTypeStr=Bus: BCE_Set
  correctionTable : Inport  Port=2  PortDimensions=[12, 4]
  Add : Sum
  Add1 : Sum
  Bus Assignment : BusAssignment  AssignedSignals=Cell_1.V,Cell_2.V,Cell_3.V,Cell_4.V,Cell_5.V,Cell_6.V,Cell_7.V,Cell_8.V,Cell_9.V,Cell_10.V,Cell_11.V,Cell_12.V,Cell_1.I,Cell_2.I,Cell_3.I,Cell_4.I,Cell_5.I,Cell_6.I,Cell_7.I,Cell_8.I,Cell_9.I,Cell_10.I,Cell_11.I,Cell_12.I
  Bus Selector : BusSelector  OutputSignals=Cell_1.V,Cell_2.V,Cell_3.V,Cell_4.V,Cell_5.V,Cell_6.V,Cell_7.V,Cell_8.V,Cell_9.V,Cell_10.V,Cell_11.V,Cell_12.V,Cell_1.I,Cell_2.I,Cell_3.I,Cell_4.I,Cell_5.I,Cell_6.I,Cell_7.I,Cell_8.I,Cell_9.I,Cell_10.I,Cell_11.I,Cell_12.I
  Data Type Conversion : DataTypeConversion  OutDataTypeStr=single  SaturateOnIntegerOverflow=off  RndMeth=Floor
  Data Type Conversion1 : DataTypeConversion  OutDataTypeStr=single  SaturateOnIntegerOverflow=off  RndMeth=Floor
  Demux : Demux  Outputs=12
  Demux1 : Demux  Outputs=12
  Product : Product
  Product1 : Product
  Selector : Selector  NumberOfDimensions=2  InputPortWidth=3  IndexOptions=Select all,Index vector (dialog)  Indices=1,1  OutputSizes=1,1
  Selector1 : Selector  NumberOfDimensions=2  InputPortWidth=3  IndexOptions=Select all,Index vector (dialog)  Indices=4,4  OutputSizes=1,1
  Selector2 : Selector  NumberOfDimensions=2  InputPortWidth=3  IndexOptions=Select all,Index vector (dialog)  Indices=2,2  OutputSizes=1,1
  Selector3 : Selector  NumberOfDimensions=2  InputPortWidth=3  IndexOptions=Select all,Index vector (dialog)  Indices=3,3  OutputSizes=1,1
  Vector Concatenate : Concatenate  NumInputs=12
  Vector Concatenate1 : Concatenate  NumInputs=12
  bceBusOut : Outport  OutDataTypeStr=Bus: BCE_Set
  wires:
  bceBusIn/1 -> Bus Selector/1, Bus Assignment/1
  correctionTable/1 -> Selector3/1, Selector1/1, Selector2/1, Selector/1
  Bus Assignment/1 -> bceBusOut/1
  Bus Selector/1 -> Vector Concatenate/1  "<V>"
  Bus Selector/2 -> Vector Concatenate/2  "<V>"
  Bus Selector/3 -> Vector Concatenate/3  "<V>"
  Bus Selector/4 -> Vector Concatenate/4  "<V>"
  Bus Selector/5 -> Vector Concatenate/5  "<V>"
  Bus Selector/6 -> Vector Concatenate/6  "<V>"
  Bus Selector/7 -> Vector Concatenate/7  "<V>"
  Bus Selector/8 -> Vector Concatenate/8  "<V>"
  Bus Selector/9 -> Vector Concatenate/9  "<V>"
  Bus Selector/10 -> Vector Concatenate/10  "<V>"
  Bus Selector/11 -> Vector Concatenate/11  "<V>"
  Bus Selector/12 -> Vector Concatenate/12  "<V>"
  Vector Concatenate/1 -> Product/2
  Product/1 -> Add/2
  Demux/7 -> Bus Assignment/8
  Demux/6 -> Bus Assignment/7
  Demux/8 -> Bus Assignment/9
  Demux/5 -> Bus Assignment/6
  Demux/9 -> Bus Assignment/10
  Demux/4 -> Bus Assignment/5
  Demux/10 -> Bus Assignment/11
  Demux/3 -> Bus Assignment/4
  Demux/11 -> Bus Assignment/12
  Demux/2 -> Bus Assignment/3
  Demux/12 -> Bus Assignment/13
  Demux/1 -> Bus Assignment/2
  Add/1 -> Data Type Conversion/1
  Add1/1 -> Data Type Conversion1/1
  Demux1/1 -> Bus Assignment/14
  Demux1/12 -> Bus Assignment/25
  Demux1/2 -> Bus Assignment/15
  Demux1/11 -> Bus Assignment/24
  Demux1/3 -> Bus Assignment/16
  Demux1/10 -> Bus Assignment/23
  Demux1/4 -> Bus Assignment/17
  Demux1/9 -> Bus Assignment/22
  Demux1/5 -> Bus Assignment/18
  Demux1/8 -> Bus Assignment/21
  Demux1/6 -> Bus Assignment/19
  Demux1/7 -> Bus Assignment/20
  Product1/1 -> Add1/2
  Vector Concatenate1/1 -> Product1/2
  Bus Selector/24 -> Vector Concatenate1/12  "<I>"
  Bus Selector/23 -> Vector Concatenate1/11  "<I>"
  Bus Selector/22 -> Vector Concatenate1/10  "<I>"
  Bus Selector/21 -> Vector Concatenate1/9  "<I>"
  Bus Selector/20 -> Vector Concatenate1/8  "<I>"
  Bus Selector/19 -> Vector Concatenate1/7  "<I>"
  Bus Selector/18 -> Vector Concatenate1/6  "<I>"
  Bus Selector/17 -> Vector Concatenate1/5  "<I>"
  Bus Selector/16 -> Vector Concatenate1/4  "<I>"
  Bus Selector/15 -> Vector Concatenate1/3  "<I>"
  Bus Selector/14 -> Vector Concatenate1/2  "<I>"
  Bus Selector/13 -> Vector Concatenate1/1  "<I>"
  Selector/1 -> [V_Gain]
  Selector2/1 -> [V_Offset]
  Selector3/1 -> [I_Gain]
  Selector1/1 -> [I_Offset]
  [V_Gain] -> Product/1
  [V_Offset] -> Add/1
  [I_Gain] -> Product1/1
  [I_Offset] -> Add1/1
  Data Type Conversion/1 -> Demux/1
  Data Type Conversion1/1 -> Demux1/1

== system speedgoatlib_bce/Templates/FIU Channel Write Template /EtherCAT State Control ==
  EC OP State : Constant  Value=8  OutDataTypeStr=int32
  EC State Compare : simulink/Logic and Bit Operations/Compare To Constant  relop=~=  const=8  OutDataTypeStr=boolean
  Get SubDevice State : slrealtimeethercatlib/Get SubDevice State  device_id=0  sample_time=1  subdevice_addr=0  selected_subdevice=Term 1 (EK1100)  timeout=500  subdevice_found=0
  Set SubDevice State : slrealtimeethercatlib/Set SubDevice State  device_id=0  sample_time=1  subdevice_addr=0  selected_subdevice=Term 1 (EK1100)  subdevice_found=0
  Terminator1 : Terminator
  Terminator2 : Terminator
  wires:
  Set SubDevice State/2 -> Terminator2/1
  EC State Compare/1 -> Set SubDevice State/2
  Set SubDevice State/1 -> Terminator1/1
  Get SubDevice State/1 -> EC State Compare/1
  EC OP State/1 -> Set SubDevice State/1

== system speedgoatlib_bce/Templates/TSE Channel Write Template /EtherCAT State Control ==
  EC OP State : Constant  Value=8  OutDataTypeStr=int32
  EC State Compare : simulink/Logic and Bit Operations/Compare To Constant  relop=~=  const=8  OutDataTypeStr=boolean
  Get SubDevice State : slrealtimeethercatlib/Get SubDevice State  device_id=0  sample_time=1  subdevice_addr=0  selected_subdevice=Term 1 (EK1100)  timeout=500  subdevice_found=0
  Set SubDevice State : slrealtimeethercatlib/Set SubDevice State  device_id=0  sample_time=1  subdevice_addr=0  selected_subdevice=Term 1 (EK1100)  subdevice_found=0
  Terminator1 : Terminator
  Terminator2 : Terminator
  wires:
  EC OP State/1 -> Set SubDevice State/1
  Get SubDevice State/1 -> EC State Compare/1
  Set SubDevice State/1 -> Terminator1/1
  EC State Compare/1 -> Set SubDevice State/2
  Set SubDevice State/2 -> Terminator2/1

== system speedgoatlib_bce/Utilities/BCE AC SM Parameter Update /Subsystem ==

== matlab function speedgoatlib_bce/Templates/FIU Channel Write Template /Range Assert ==
  data: u input; y output
function y = fcn(u)

    y = sg_bce.fiuFaultStateRangeAssert(u);

end

== matlab function speedgoatlib_bce/Templates/BCE AC SM Parameter Update Template /MATLAB Function ==
  data: SeqTimeStep input uint16 size=[1,12]; cell output uint16 size=[12,14]; SeqTimeUnit input boolean size=[1,12]; SeqOutputPath input boolean size=[1,12]; SeqStartDelay input uint16 size=[1,12]; SeqNumCycles input uint16 size=[1,12]; SeqGainAdjustment input double size=[1,12]; SeqGainSweepEnable input boolean size=[1,12]; SeqTimeSweepEnable input boolean size=[1,12]; SeqGainSweepUpdateTime input uint16 size=[1,12]; SeqTimeSweepUpdateTime input uint16 size=[1,12]; SeqGainSweepUpdateStep input double size=[1,12]; SeqTimeSweepUpdateStep input uint16 size=[1,12]; SeqGainSweepLimitValue input double size=[1,12]; SeqTimeSweepLimitValue input uint16 size=[1,12]
function cell = fcn(SeqTimeStep,SeqTimeUnit,SeqOutputPath,SeqStartDelay,SeqNumCycles, ...
        SeqGainAdjustment,SeqGainSweepEnable,SeqTimeSweepEnable,SeqGainSweepUpdateTime, ...
        SeqTimeSweepUpdateTime,SeqGainSweepUpdateStep,SeqTimeSweepUpdateStep, ...
        SeqGainSweepLimitValue,SeqTimeSweepLimitValue)

    numCells = 12;
    numSeqIndices = 13;
    cell = zeros(numCells, numSeqIndices+1, 'uint16');

    cell = sg_bce.prepareSequencerParams(SeqTimeStep,SeqTimeUnit,SeqOutputPath,SeqStartDelay,SeqNumCycles, ...
            SeqGainAdjustment,SeqGainSweepEnable,SeqTimeSweepEnable,SeqGainSweepUpdateTime, ...
            SeqTimeSweepUpdateTime,SeqGainSweepUpdateStep,SeqTimeSweepUpdateStep, ...
            SeqGainSweepLimitValue,SeqTimeSweepLimitValue);

end
